simulink model "gm_rgb_gauss_sobel_64bit_full"  (R2022a)
settings: Solver=VariableStepAuto  StartTime=0.0  StopTime=10.0  RelTol=1e-3
undefined symbols (not defined in the file or in its folder): blueMax, blueMin, gray, greenMax, greenMin, redMax, redMin
libraries: hdlsllib x62, visionhdlio x6, visionsources x2
(part 1 of 3)
settings Model: PacingRate=1000  Creator=cxc1831  LastModifiedBy=calvi
settings OptimizationCC: BlockReduction=off  ConditionallyExecuteInputs=off
settings DebuggingCC: ArtificialAlgebraicLoopMsg=none  InheritedTsInSrcMsg=none

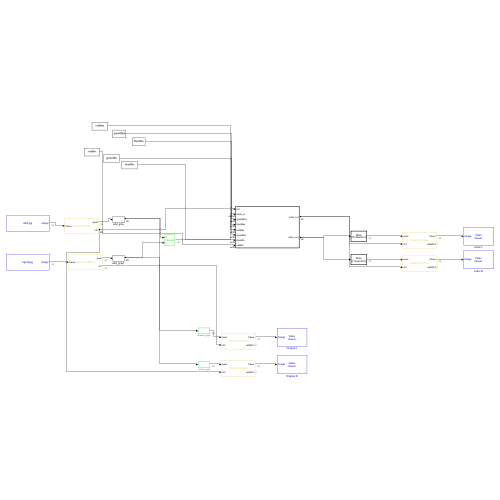
[thumbnail: Simulink's stored preview of the top-level diagram]
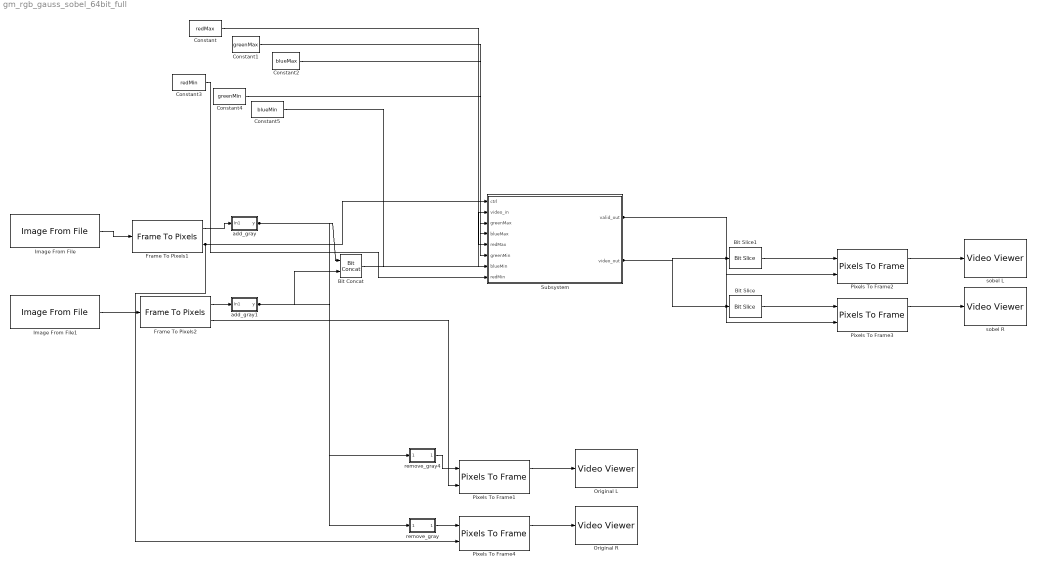
== system gm_rgb_gauss_sobel_64bit_full ==
  Bit Concat : hdlsllib/Logic and Bit Operations/Bit Concat  numInputs=2
  Bit Slice : hdlsllib/Logic and Bit Operations/Bit Slice  lidx=7  ridx=0
      settings: SourceProductBaseCode=SL
  Bit Slice1 : hdlsllib/Logic and Bit Operations/Bit Slice  lidx=15  ridx=8
      settings: SourceProductBaseCode=SL
  Constant : Constant  Value=redMax  OutDataTypeStr=uint8  SampleTime=-1
  Constant1 : Constant  Value=greenMax  OutDataTypeStr=uint8  SampleTime=-1
  Constant2 : Constant  Value=blueMax  OutDataTypeStr=uint8  SampleTime=-1
  Constant3 : Constant  Value=redMin  OutDataTypeStr=uint8  SampleTime=-1  LockScale=on
  Constant4 : Constant  Value=greenMin  OutDataTypeStr=uint8  SampleTime=-1  LockScale=on
  Constant5 : Constant  Value=blueMin  OutDataTypeStr=uint8  SampleTime=-1  LockScale=on
  Frame To Pixels1 : visionhdlio/Frame To Pixels  NumComponents=3  NumPixels=1  VideoFormat=Custom  ActivePixelsPerLine=R  ActiveVideoLines=C  TotalPixelsPerLine=R  TotalVideoLines=C  StartingActiveLine=1  FrontPorch=0  SampleTime=0  VideoFormatCache=Custom  ActivePixelsPerLineCache=R  ActiveVideoLinesCache=C  TotalPixelsPerLineCache=R  TotalVideoLinesCache=C  StartingActiveLineCache=1  FrontPorchCache=0
      settings: SourceProductBaseCode=VT
  Frame To Pixels2 : visionhdlio/Frame To Pixels  NumComponents=3  NumPixels=1  VideoFormat=Custom  ActivePixelsPerLine=R  ActiveVideoLines=C  TotalPixelsPerLine=R  TotalVideoLines=C  StartingActiveLine=1  FrontPorch=0  SampleTime=0  VideoFormatCache=Custom  ActivePixelsPerLineCache=R  ActiveVideoLinesCache=C  TotalPixelsPerLineCache=R  TotalVideoLinesCache=C  StartingActiveLineCache=1  FrontPorchCache=0
      settings: SourceProductBaseCode=VT
  Image From File : visionsources/Image From File  Tag=vipblks_nd  FileName=C:\Projects\ipcore_integration\left3.jpg  Ts=1  imagePorts=One multidimensional signal  OutPortLabels=R|G|B  ImageDataType=Inherit from input image  sdImageDataType=uint(8)  Signed=on  WordLength=16  FractionLengthMode=User-defined  FractionLength=15
  Image From File1 : visionsources/Image From File  Tag=vipblks_nd  FileName=C:\Projects\ipcore_integration\right3.jpg  Ts=1  imagePorts=One multidimensional signal  OutPortLabels=R|G|B  ImageDataType=Inherit from input image  sdImageDataType=uint(8)  Signed=on  WordLength=16  FractionLengthMode=User-defined  FractionLength=15
  Original L : VideoViewer  colormapValue=gray(256)  FigPos=[661 769 562 322]
  Original R : VideoViewer  colormapValue=gray(256)  FigPos=[692 754 485 298]
  Pixels To Frame1 : visionhdlio/Pixels To Frame  NumComponents=3  NumPixels=1  VideoFormat=Custom  ActivePixelsPerLine=R  ActiveVideoLines=C  TotalPixelsPerLine=R  TotalVideoLines=C  VideoFormatCache=Custom  ActivePixelsPerLineCache=R  ActiveVideoLinesCache=C  TotalPixelsPerLineCache=R  TotalVideoLinesCache=C
      settings: SourceProductBaseCode=VT
  Pixels To Frame2 : visionhdlio/Pixels To Frame  NumComponents=1  NumPixels=1  VideoFormat=Custom  ActivePixelsPerLine=R  ActiveVideoLines=C  TotalPixelsPerLine=R  TotalVideoLines=C  VideoFormatCache=Custom  ActivePixelsPerLineCache=R  ActiveVideoLinesCache=C  TotalPixelsPerLineCache=R  TotalVideoLinesCache=C
      settings: SourceProductBaseCode=VT
  Pixels To Frame3 : visionhdlio/Pixels To Frame  NumComponents=1  NumPixels=1  VideoFormat=Custom  ActivePixelsPerLine=R  ActiveVideoLines=C  TotalPixelsPerLine=R  TotalVideoLines=C  VideoFormatCache=Custom  ActivePixelsPerLineCache=R  ActiveVideoLinesCache=C  TotalPixelsPerLineCache=R  TotalVideoLinesCache=C
      settings: SourceProductBaseCode=VT
  Pixels To Frame4 : visionhdlio/Pixels To Frame  NumComponents=3  NumPixels=1  VideoFormat=Custom  ActivePixelsPerLine=R  ActiveVideoLines=C  TotalPixelsPerLine=R  TotalVideoLines=C  VideoFormatCache=Custom  ActivePixelsPerLineCache=R  ActiveVideoLinesCache=C  TotalPixelsPerLineCache=R  TotalVideoLinesCache=C
      settings: SourceProductBaseCode=VT
  Subsystem : Subsystem  TreatAsAtomicUnit=on
  add_gray : Subsystem
  add_gray1 : Subsystem
  remove_gray : Subsystem
  remove_gray4 : Subsystem
  sobel L : VideoViewer  colormapValue=gray(256)  FigPos=[1 1398 2560 1298]
  sobel R : VideoViewer  colormapValue=gray(256)  FigPos=[1 1398 2560 1298]
  wires:
  Constant5/1 -> Subsystem/7(blueMin)
  Constant4/1 -> Subsystem/6(greenMin)
  Constant3/1 -> Subsystem/8(redMin)
  Constant2/1 -> Subsystem/4(blueMax)
  Constant/1 -> Subsystem/5(redMax)
  Constant1/1 -> Subsystem/3(greenMax)
  Subsystem/1(valid_out) -> Pixels To Frame2/2, Pixels To Frame3/2
  Subsystem/2(video_out) -> Bit Slice/1, Bit Slice1/1
  Bit Concat/1 -> Subsystem/2(video_in)
  Bit Slice1/1 -> Pixels To Frame2/1
  Bit Slice/1 -> Pixels To Frame3/1
  Pixels To Frame3/1 -> sobel R/1
  Pixels To Frame2/1 -> sobel L/1
  Pixels To Frame4/1 -> Original R/1
  Pixels To Frame1/1 -> Original L/1
  Frame To Pixels2/1 -> add_gray1/1(In1)
  Frame To Pixels1/1 -> add_gray/1(In1)
  Image From File/1 -> Frame To Pixels1/1
  add_gray1/1(y) -> Bit Concat/2, remove_gray/1(RGB)
  Frame To Pixels1/2 -> Pixels To Frame4/2, Subsystem/1(ctrl)
  remove_gray/1(RGBVector) -> Pixels To Frame4/1
  Image From File1/1 -> Frame To Pixels2/1
  add_gray/1(y) -> Bit Concat/1, remove_gray4/1(RGB)
  remove_gray4/1(RGBVector) -> Pixels To Frame1/1
  Frame To Pixels2/2 -> Pixels To Frame1/2

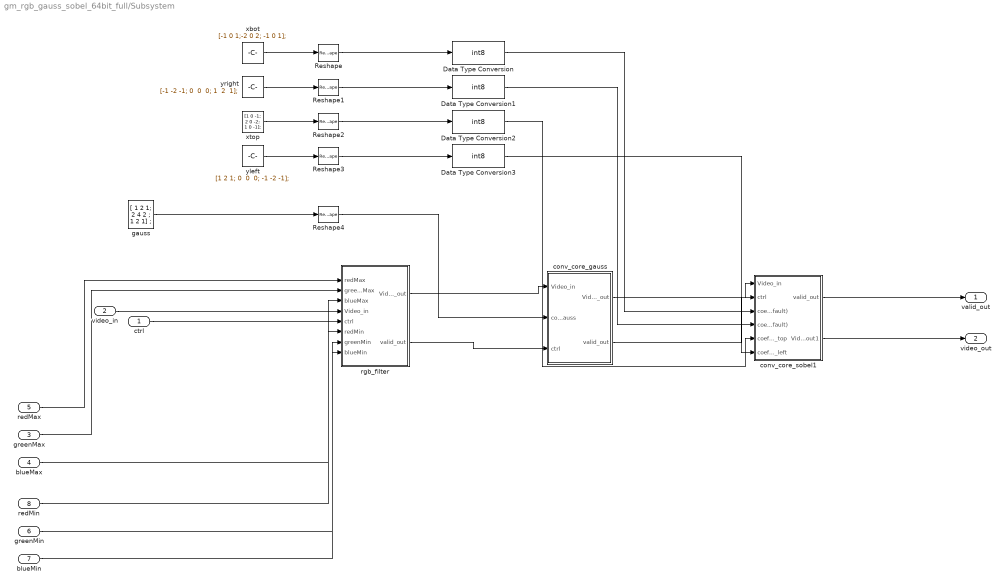
== system gm_rgb_gauss_sobel_64bit_full/Subsystem ==
  ctrl : Inport  SampleTime=2.77039007092199e-06
  video_in : Inport  Port=2  OutDataTypeStr=fixdt(0, 64, 0)  PortDimensions=1  SampleTime=2.77039007092199e-06
  greenMax : Inport  Port=3  OutDataTypeStr=uint8  PortDimensions=1  SampleTime=2.77039007092199e-06
  blueMax : Inport  Port=4  OutDataTypeStr=uint8  PortDimensions=1  SampleTime=2.77039007092199e-06
  redMax : Inport  Port=5  OutDataTypeStr=uint8  PortDimensions=1  SampleTime=2.77039007092199e-06
  greenMin : Inport  Port=6  OutDataTypeStr=uint8  PortDimensions=1  SampleTime=2.77039007092199e-06
  blueMin : Inport  Port=7  OutDataTypeStr=uint8  PortDimensions=1  SampleTime=2.77039007092199e-06
  redMin : Inport  Port=8  OutDataTypeStr=uint8  PortDimensions=1  SampleTime=2.77039007092199e-06
  Data Type Conversion{,1..3} (4 alike) : DataTypeConversion  OutDataTypeStr=int8  SaturateOnIntegerOverflow=off  RndMeth=Floor
  Reshape{,1..4} (5 alike) : Reshape
  conv_core_gauss : Subsystem
  conv_core_sobel1 : Subsystem
  gauss : Constant  Value=|  VectorParams1D=off  OutDataTypeStr=uint8  SampleTime=-1  LockScale=on
      | [ 1  2  1;  2   4   2 ;  1  2  1]
      | ;
  rgb_filter : Subsystem
  xbot : Constant  Value=|  VectorParams1D=off  OutDataTypeStr=int8  SampleTime=-1
      | [-1 0 1;-2 0 2;
      | -1 0 1];
  xtop : Constant  Value=|  VectorParams1D=off  OutDataTypeStr=int8  SampleTime=-1
      | [1 0 -1; 2 0 -2;
      | 1 0 -1];
  yleft : Constant  Value="[1 2 1; 0  0  0; -1 -2 -1];"  VectorParams1D=off  OutDataTypeStr=int8  SampleTime=-1
  yright : Constant  Value=|  VectorParams1D=off  OutDataTypeStr=int8  SampleTime=-1
      | [-1 -2 -1;
      | 0  0  0; 1  2  1];
  valid_out : Outport  SampleTime=2.77039007092199e-06
  video_out : Outport  Port=2  SampleTime=2.77039007092199e-06
  wires:
  ctrl/1 -> rgb_filter/5(ctrl)
  video_in/1 -> rgb_filter/4(Video_in)
  greenMax/1 -> rgb_filter/2(greenMax)
  blueMax/1 -> rgb_filter/3(blueMax)
  redMax/1 -> rgb_filter/1(redMax)
  greenMin/1 -> rgb_filter/7(greenMin)
  blueMin/1 -> rgb_filter/8(blueMin)
  redMin/1 -> rgb_filter/6(redMin)
  Data Type Conversion/1 -> conv_core_sobel1/3(coeffsX_bot(default))
  Data Type Conversion1/1 -> conv_core_sobel1/4(coeffsY_right(default))
  Data Type Conversion2/1 -> conv_core_sobel1/5(coeffsX_top)
  Data Type Conversion3/1 -> conv_core_sobel1/6(coeffsY_left)
  Reshape/1 -> Data Type Conversion/1
  Reshape1/1 -> Data Type Conversion1/1
  Reshape2/1 -> Data Type Conversion2/1
  Reshape3/1 -> Data Type Conversion3/1
  Reshape4/1 -> conv_core_gauss/2(coeffsGauss)
  conv_core_gauss/1(Video_out) -> conv_core_sobel1/1(Video_in)
  conv_core_gauss/2(valid_out) -> conv_core_sobel1/2(ctrl)
  conv_core_sobel1/1(valid_out) -> valid_out/1
  conv_core_sobel1/2(Video_out1) -> video_out/1
  gauss/1 -> Reshape4/1
  rgb_filter/1(Video_out) -> conv_core_gauss/1(Video_in)
  rgb_filter/2(valid_out) -> conv_core_gauss/3(ctrl)
  xbot/1 -> Reshape/1
  xtop/1 -> Reshape2/1
  yleft/1 -> Reshape3/1
  yright/1 -> Reshape1/1

== system gm_rgb_gauss_sobel_64bit_full/add_gray ==
  note: Grayscale = (R * 0.25) + (G * 0.5) + (B * 0.125)
  In1 : Inport
  Bit Concat : hdlsllib/Logic and Bit Operations/Bit Concat  numInputs=4
  Demux : Demux  Outputs=3
  Shift Arithmetic3 : ArithShift  BitShiftNumber=1  BitShiftDirection=Right
  Shift Arithmetic4 : ArithShift  BitShiftNumber=2  BitShiftDirection=Right
  Shift Arithmetic5 : ArithShift  BitShiftNumber=3  BitShiftDirection=Right
  Sum : Sum  Inputs=+++  OutDataTypeStr=uint8
  y : Outport
  wires:
  Shift Arithmetic5/1 -> Sum/3
  Shift Arithmetic3/1 -> Sum/2
  Shift Arithmetic4/1 -> Sum/1
  Sum/1 -> Bit Concat/1
  Demux/3 -> Bit Concat/4, Shift Arithmetic5/1
  Demux/1 -> Bit Concat/2, Shift Arithmetic4/1
  Demux/2 -> Bit Concat/3, Shift Arithmetic3/1
  In1/1 -> Demux/1
  Bit Concat/1 -> y/1

== system gm_rgb_gauss_sobel_64bit_full/add_gray1 ==
  note: Grayscale = (R * 0.25) + (G * 0.5) + (B * 0.125)
  In1 : Inport
  Bit Concat : hdlsllib/Logic and Bit Operations/Bit Concat  numInputs=4
  Demux : Demux  Outputs=3
  Shift Arithmetic3 : ArithShift  BitShiftNumber=1  BitShiftDirection=Right
  Shift Arithmetic4 : ArithShift  BitShiftNumber=2  BitShiftDirection=Right
  Shift Arithmetic5 : ArithShift  BitShiftNumber=3  BitShiftDirection=Right
  Sum : Sum  Inputs=+++  OutDataTypeStr=uint8
  y : Outport
  wires:
  Shift Arithmetic5/1 -> Sum/3
  Shift Arithmetic3/1 -> Sum/2
  Shift Arithmetic4/1 -> Sum/1
  Sum/1 -> Bit Concat/1
  Demux/3 -> Bit Concat/4, Shift Arithmetic5/1
  Demux/1 -> Bit Concat/2, Shift Arithmetic4/1
  Demux/2 -> Bit Concat/3, Shift Arithmetic3/1
  In1/1 -> Demux/1
  Bit Concat/1 -> y/1

== system gm_rgb_gauss_sobel_64bit_full/remove_gray ==
  note: RGB represented in
      | 32'hFFRRGGBB
  RGB : Inport
  Bit Slice : hdlsllib/Logic and Bit Operations/Bit Slice  lidx=23  ridx=16
      settings: SourceProductBaseCode=SL
  Bit Slice1 : hdlsllib/Logic and Bit Operations/Bit Slice  lidx=15  ridx=8
      settings: SourceProductBaseCode=SL
  Bit Slice2 : hdlsllib/Logic and Bit Operations/Bit Slice  lidx=7  ridx=0
      settings: SourceProductBaseCode=SL
  Mux : Mux  Inputs=3
  Signal Specification : SignalSpecification
  Transpose : Math  Operator=transpose  SignedPower=on
  RGBVector : Outport  VectorParamsAs1DForOutWhenUnconnected=off
  wires:
  Mux/1 -> Transpose/1
  Bit Slice/1 -> Mux/1
  Bit Slice2/1 -> Mux/3
  Bit Slice1/1 -> Mux/2
  RGB/1 -> Bit Slice2/1, Bit Slice1/1, Bit Slice/1
  Transpose/1 -> Signal Specification/1
  Signal Specification/1 -> RGBVector/1

== system gm_rgb_gauss_sobel_64bit_full/remove_gray4 ==
  note: RGB represented in
      | 32'hFFRRGGBB
  RGB : Inport
  Bit Slice : hdlsllib/Logic and Bit Operations/Bit Slice  lidx=23  ridx=16
      settings: SourceProductBaseCode=SL
  Bit Slice1 : hdlsllib/Logic and Bit Operations/Bit Slice  lidx=15  ridx=8
      settings: SourceProductBaseCode=SL
  Bit Slice2 : hdlsllib/Logic and Bit Operations/Bit Slice  lidx=7  ridx=0
      settings: SourceProductBaseCode=SL
  Mux : Mux  Inputs=3
  Signal Specification : SignalSpecification
  Transpose : Math  Operator=transpose  SignedPower=on
  RGBVector : Outport  VectorParamsAs1DForOutWhenUnconnected=off
  wires:
  Mux/1 -> Transpose/1
  Bit Slice/1 -> Mux/1
  Bit Slice2/1 -> Mux/3
  Bit Slice1/1 -> Mux/2
  RGB/1 -> Bit Slice2/1, Bit Slice1/1, Bit Slice/1
  Transpose/1 -> Signal Specification/1
  Signal Specification/1 -> RGBVector/1

== system gm_rgb_gauss_sobel_64bit_full/Subsystem/conv_core_gauss ==
  Video_in : Inport  OutDataTypeStr=fixdt(0, 64, 0)  PortDimensions=1  SampleTime=2.77039007092199e-06
  coeffsGauss : Inport  Port=2  OutDataTypeStr=uint8  PortDimensions=[9]  SampleTime=2.77039007092199e-06
  ctrl : Inport  Port=3  SampleTime=2.77039007092199e-06
  Bus Selector : BusSelector  OutputSignals=valid
  Delay1 : Delay  InitialCondition=0
  Subsystem1 : Subsystem
  Video_out : Outport  SampleTime=2.77039007092199e-06  VectorParamsAs1DForOutWhenUnconnected=off
  valid_out : Outport  Port=2  SampleTime=2.77039007092199e-06  VectorParamsAs1DForOutWhenUnconnected=off
  wires:
  Video_in/1 -> Subsystem1/1(VideoIn)
  coeffsGauss/1 -> Subsystem1/2(coeffsGauss)
  ctrl/1 -> Bus Selector/1, Delay1/1
  Bus Selector/1 -> Subsystem1/3(Enable)
  Delay1/1 -> valid_out/1
  Subsystem1/1(Video_out) -> Video_out/1

== system gm_rgb_gauss_sobel_64bit_full/Subsystem/conv_core_sobel1 ==
  Video_in : Inport  OutDataTypeStr=fixdt(0, 64, 0)  PortDimensions=1  SampleTime=2.77039007092199e-06
  ctrl : Inport  Port=2  SampleTime=2.77039007092199e-06
  coeffsX_bot(default) : Inport  Port=3  OutDataTypeStr=int8  PortDimensions=[9]  SampleTime=2.77039007092199e-06
  coeffsY_right(default) : Inport  Port=4  OutDataTypeStr=int8  PortDimensions=[9]  SampleTime=2.77039007092199e-06
  coeffsX_top : Inport  Port=5  OutDataTypeStr=int8  PortDimensions=[9]  SampleTime=2.77039007092199e-06
  coeffsY_left : Inport  Port=6  OutDataTypeStr=int8  PortDimensions=[9]  SampleTime=2.77039007092199e-06
  Bit Concat1 : hdlsllib/Logic and Bit Operations/Bit Concat  numInputs=2
  Bus Selector : BusSelector  OutputSignals=valid
  Delay1 : Delay  InitialCondition=0
  Subsystem1 : Subsystem
  valid_out : Outport  SampleTime=2.77039007092199e-06  VectorParamsAs1DForOutWhenUnconnected=off
  Video_out1 : Outport  Port=2  SampleTime=2.77039007092199e-06  VectorParamsAs1DForOutWhenUnconnected=off
  wires:
  Video_in/1 -> Subsystem1/1(vidIn)
  ctrl/1 -> Bus Selector/1, Delay1/1
  coeffsX_bot(default)/1 -> Subsystem1/2(coeffsX_bot(default))
  coeffsY_right(default)/1 -> Subsystem1/3(coeffsY_bot(default))
  coeffsX_top/1 -> Subsystem1/4(coeffsX_Top)
  coeffsY_left/1 -> Subsystem1/5(coeffsY_Left)
  Bit Concat1/1 -> Video_out1/1
  Bus Selector/1 -> Subsystem1/6(Enable)
  Delay1/1 -> valid_out/1
  Subsystem1/1(sobel R) -> Bit Concat1/2
  Subsystem1/2(sobel L) -> Bit Concat1/1

== system gm_rgb_gauss_sobel_64bit_full/Subsystem/rgb_filter ==
  redMax : Inport  OutDataTypeStr=uint8  PortDimensions=1  SampleTime=2.77039007092199e-06
  greenMax : Inport  Port=2  OutDataTypeStr=uint8  PortDimensions=1  SampleTime=2.77039007092199e-06
  blueMax : Inport  Port=3  OutDataTypeStr=uint8  PortDimensions=1  SampleTime=2.77039007092199e-06
  Video_in : Inport  Port=4  OutDataTypeStr=fixdt(0, 64, 0)  PortDimensions=1  SampleTime=2.77039007092199e-06
  ctrl : Inport  Port=5  SampleTime=2.77039007092199e-06
  redMin : Inport  Port=6  OutDataTypeStr=uint8  PortDimensions=1  SampleTime=2.77039007092199e-06
  greenMin : Inport  Port=7  OutDataTypeStr=uint8  PortDimensions=1  SampleTime=2.77039007092199e-06
  blueMin : Inport  Port=8  OutDataTypeStr=uint8  PortDimensions=1  SampleTime=2.77039007092199e-06
  Bit Concat1 : hdlsllib/Logic and Bit Operations/Bit Concat  numInputs=2
  Bus Selector : BusSelector  OutputSignals=valid
  Delay1 : Delay  DelayLength=1  InitialCondition=0
  Subsystem1 : Subsystem
  Video_out : Outport  SampleTime=2.77039007092199e-06  VectorParamsAs1DForOutWhenUnconnected=off
  valid_out : Outport  Port=2  SampleTime=2.77039007092199e-06  VectorParamsAs1DForOutWhenUnconnected=off
  wires:
  redMax/1 -> Subsystem1/2(redmax)
  greenMax/1 -> Subsystem1/3(greenmax)
  blueMax/1 -> Subsystem1/4(bluemax)
  Video_in/1 -> Subsystem1/1(In2)
  ctrl/1 -> Bus Selector/1, Delay1/1
  redMin/1 -> Subsystem1/5(redMin)
  greenMin/1 -> Subsystem1/6(greenMin)
  blueMin/1 -> Subsystem1/7(blueMin)
  Bit Concat1/1 -> Video_out/1
  Bus Selector/1 -> Subsystem1/8(Enable)
  Delay1/1 -> valid_out/1
  Subsystem1/1(Video_outLeft) -> Bit Concat1/1
  Subsystem1/2(Video_outRight) -> Bit Concat1/2

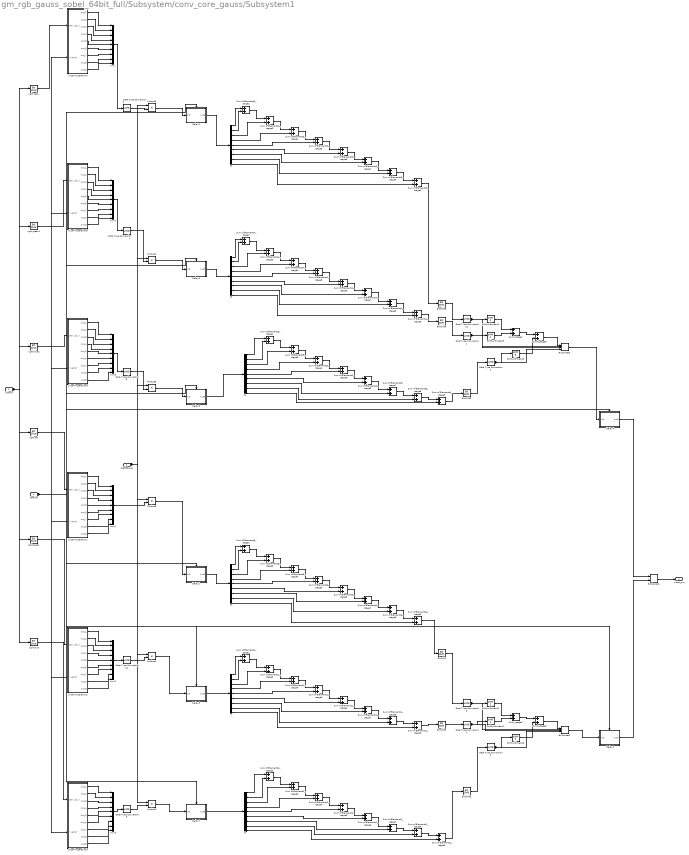
== system gm_rgb_gauss_sobel_64bit_full/Subsystem/conv_core_gauss/Subsystem1 ==
  VideoIn : Inport  OutDataTypeStr=fixdt(0, 64, 0)  PortDimensions=1  SampleTime=2.77039007092199e-06
  coeffsGauss : Inport  Port=2  OutDataTypeStr=uint8  PortDimensions=[9]  SampleTime=2.77039007092199e-06
  Enable : Inport  Port=3  OutDataTypeStr=boolean  SampleTime=2.77039007092199e-06
  Bit Concat1 : hdlsllib/Logic and Bit Operations/Bit Concat  numInputs=2
  Bit Concat2 : hdlsllib/Logic and Bit Operations/Bit Concat  numInputs=4
  Bit Concat3 : hdlsllib/Logic and Bit Operations/Bit Concat  numInputs=4
  Bit Shift{,1..5} (6 alike) : hdlsllib/Logic and Bit Operations/Bit Shift  mode=Shift Right Arithmetic  N=double(4)
  Data Type Conversion{1..10,12} (11 alike) : DataTypeConversion  OutDataTypeStr=uint8  SampleTime=2.77039007092199e-06  SaturateOnIntegerOverflow=off  RndMeth=Floor
  Delay1 : Subsystem
      settings: MinAlgLoopOccurrences=on
  Delay2 : Subsystem
      settings: MinAlgLoopOccurrences=on
  Delay3 : Subsystem
      settings: MinAlgLoopOccurrences=on
  Delay4 : Subsystem
      settings: MinAlgLoopOccurrences=on
  Delay5 : Subsystem
      settings: MinAlgLoopOccurrences=on
  Delay6 : Subsystem
      settings: MinAlgLoopOccurrences=on
  Delay7 : Subsystem
      settings: MinAlgLoopOccurrences=on
  Delay8 : Subsystem
      settings: MinAlgLoopOccurrences=on
  Product{1..6} (6 alike) : Product  Inputs=**  OutDataTypeStr=uint16  SaturateOnIntegerOverflow=on  SampleTime=2.77039007092199e-06
  Shift Arithmetic1 : ArithShift  BitShiftNumber=1  BinPtShiftNumber=double(0)
  Shift Arithmetic2 : ArithShift  BitShiftNumber=2  BinPtShiftNumber=double(0)
  Shift Arithmetic3 : ArithShift  BitShiftNumber=1  BinPtShiftNumber=double(0)
  Shift Arithmetic4 : ArithShift  BitShiftNumber=2  BinPtShiftNumber=double(0)
  Shift Arithmetic5 : ArithShift  BitShiftNumber=3  BinPtShiftNumber=double(0)
  Shift Arithmetic6 : ArithShift  BitShiftNumber=3  BinPtShiftNumber=double(0)
  Sum of Elements1_stage{2..9} (8 alike) : Sum  AccumDataTypeStr=uint32  OutDataTypeStr=uint32  SaturateOnIntegerOverflow=on  SampleTime=2.77039007092199e-06
  Sum of Elements2_stage{2..9} (8 alike) : Sum  AccumDataTypeStr=uint32  OutDataTypeStr=uint32  SaturateOnIntegerOverflow=on  SampleTime=2.77039007092199e-06
  Sum of Elements3_stage{2..9} (8 alike) : Sum  AccumDataTypeStr=uint32  OutDataTypeStr=uint32  SaturateOnIntegerOverflow=on  SampleTime=2.77039007092199e-06
  Sum of Elements4_stage{2..9} (8 alike) : Sum  AccumDataTypeStr=uint32  OutDataTypeStr=uint32  SaturateOnIntegerOverflow=on  SampleTime=2.77039007092199e-06
  Sum of Elements5_stage{2..9} (8 alike) : Sum  AccumDataTypeStr=uint32  OutDataTypeStr=uint32  SaturateOnIntegerOverflow=on  SampleTime=2.77039007092199e-06
  Sum of Elements6_stage{2..9} (8 alike) : Sum  AccumDataTypeStr=uint32  OutDataTypeStr=uint32  SaturateOnIntegerOverflow=on  SampleTime=2.77039007092199e-06
  Sum1_stage2 : Sum  AccumDataTypeStr=uint8  OutDataTypeStr=uint8  SampleTime=2.77039007092199e-06
  Sum1_stage3 : Sum  AccumDataTypeStr=uint8  OutDataTypeStr=uint8  SampleTime=2.77039007092199e-06
  Sum2_stage2 : Sum  AccumDataTypeStr=uint8  OutDataTypeStr=uint8  SampleTime=2.77039007092199e-06
  Sum2_stage3 : Sum  AccumDataTypeStr=uint8  OutDataTypeStr=uint8  SampleTime=2.77039007092199e-06
  mux{,1..5} (6 alike) : Mux  Inputs=9
  right blue : hdlsllib/Logic and Bit Operations/Bit Slice  lidx=double(7)  ridx=double(0)
      settings: SourceProductBaseCode=SL
  right blue1 : hdlsllib/Logic and Bit Operations/Bit Slice  lidx=double(39)  ridx=double(32)
      settings: SourceProductBaseCode=SL
  right green : hdlsllib/Logic and Bit Operations/Bit Slice  lidx=double(15)  ridx=double(8)
      settings: SourceProductBaseCode=SL
  right green1 : hdlsllib/Logic and Bit Operations/Bit Slice  lidx=double(47)  ridx=double(40)
      settings: SourceProductBaseCode=SL
  right red : hdlsllib/Logic and Bit Operations/Bit Slice  lidx=double(23)  ridx=double(16)
      settings: SourceProductBaseCode=SL
  right red1 : hdlsllib/Logic and Bit Operations/Bit Slice  lidx=double(55)  ridx=double(48)
      settings: SourceProductBaseCode=SL
  slicer R operation1 : Subsystem
  slicer R operation2 : Subsystem
  slicer R operation3 : Subsystem
  slicer R operation4 : Subsystem
  slicer R operation5 : Subsystem
  slicer R operation6 : Subsystem
  t{,1..5} (6 alike) : Demux  Outputs=9
  Video_out : Outport  SampleTime=2.77039007092199e-06  InitialOutput=0  VectorParamsAs1DForOutWhenUnconnected=off
  wires:
  Enable/1 -> Delay8/Enable, Delay7/Enable, Delay6/Enable, Delay5/Enable, Delay4/Enable, Delay3/Enable, Delay2/Enable, Delay1/Enable, slicer R operation6/2(<valid>), slicer R operation5/2(<valid>), slicer R operation4/2(<valid>), slicer R operation3/2(<valid>), slicer R operation2/2(<valid>), slicer R operation1/2(<valid>)
  VideoIn/1 -> right red1/1, right red/1, right green1/1, right green/1, right blue1/1, right blue/1
  coeffsGauss/1 -> Product6/1, Product5/1, Product4/1, Product3/1, Product2/1, Product1/1
  Bit Concat1/1 -> Video_out/1
  Bit Concat2/1 -> Delay3/1(in0)
  Bit Concat3/1 -> Delay4/1(in0)
  Bit Shift/1 -> Data Type Conversion5/1
  Bit Shift1/1 -> Data Type Conversion4/1
  Bit Shift2/1 -> Data Type Conversion3/1
  Bit Shift3/1 -> Data Type Conversion12/1
  Bit Shift4/1 -> Data Type Conversion1/1
  Bit Shift5/1 -> Data Type Conversion2/1
  Data Type Conversion1/1 -> Shift Arithmetic3/1, Bit Concat3/3
  Data Type Conversion10/1 -> Product1/2
  Data Type Conversion12/1 -> Shift Arithmetic4/1, Bit Concat3/2
  Data Type Conversion2/1 -> Shift Arithmetic5/1, Bit Concat3/4
  Data Type Conversion3/1 -> Shift Arithmetic6/1, Bit Concat2/4
  Data Type Conversion4/1 -> Shift Arithmetic1/1, Bit Concat2/3
  Data Type Conversion5/1 -> Shift Arithmetic2/1, Bit Concat2/2
  Data Type Conversion6/1 -> Product3/2
  Data Type Conversion7/1 -> Product4/2
  Data Type Conversion8/1 -> Product5/2
  Data Type Conversion9/1 -> Product2/2
  Delay1/1(out0) -> t5/1
  Delay2/1(out0) -> t2/1
  Delay3/1(out0) -> Bit Concat1/2
  Delay4/1(out0) -> Bit Concat1/1
  Delay5/1(out0) -> t/1
  Delay6/1(out0) -> t3/1
  Delay7/1(out0) -> t1/1
  Delay8/1(out0) -> t4/1
  mux/1 -> Data Type Conversion6/1
  mux1/1 -> Product6/2
  mux2/1 -> Data Type Conversion10/1
  mux3/1 -> Data Type Conversion9/1
  mux4/1 -> Data Type Conversion7/1
  mux5/1 -> Data Type Conversion8/1
  Product1/1 -> Delay5/1(in0)
  Product2/1 -> Delay7/1(in0)
  Product3/1 -> Delay2/1(in0)
  Product4/1 -> Delay6/1(in0)
  Product5/1 -> Delay8/1(in0)
  Product6/1 -> Delay1/1(in0)
  Shift Arithmetic1/1 -> Sum1_stage2/2
  Shift Arithmetic2/1 -> Sum1_stage2/1
  Shift Arithmetic3/1 -> Sum2_stage2/2
  Shift Arithmetic4/1 -> Sum2_stage2/1
  Shift Arithmetic5/1 -> Sum2_stage3/2
  Shift Arithmetic6/1 -> Sum1_stage3/2
  Sum1_stage3/1 -> Bit Concat2/1
  Sum2_stage3/1 -> Bit Concat3/1
  right blue/1 -> slicer R operation3/1(channel_in)
  right blue1/1 -> slicer R operation6/1(channel_in)
  right green/1 -> slicer R operation2/1(channel_in)
  right green1/1 -> slicer R operation5/1(channel_in)
  right red/1 -> slicer R operation1/1(channel_in)
  right red1/1 -> slicer R operation4/1(channel_in)
  slicer R operation1/1(out_1) -> mux1/1
  slicer R operation1/2(out_2) -> mux1/2
  slicer R operation1/3(out_3) -> mux1/3
  slicer R operation1/4(out_4) -> mux1/4
  slicer R operation1/5(out_5) -> mux1/5
  slicer R operation1/6(out_6) -> mux1/6
  slicer R operation1/7(out_7) -> mux1/7
  slicer R operation1/8(out_8) -> mux1/8
  slicer R operation1/9(out_9) -> mux1/9
  slicer R operation2/1(out_1) -> mux2/1
  slicer R operation2/2(out_2) -> mux2/2
  slicer R operation2/3(out_3) -> mux2/3
  slicer R operation2/4(out_4) -> mux2/4
  slicer R operation2/5(out_5) -> mux2/5
  slicer R operation2/6(out_6) -> mux2/6
  slicer R operation2/7(out_7) -> mux2/7
  slicer R operation2/8(out_8) -> mux2/8
  slicer R operation2/9(out_9) -> mux2/9
  slicer R operation3/1(out_1) -> mux3/1
  slicer R operation3/2(out_2) -> mux3/2
  slicer R operation3/3(out_3) -> mux3/3
  slicer R operation3/4(out_4) -> mux3/4
  slicer R operation3/5(out_5) -> mux3/5
  slicer R operation3/6(out_6) -> mux3/6
  slicer R operation3/7(out_7) -> mux3/7
  slicer R operation3/8(out_8) -> mux3/8
  slicer R operation3/9(out_9) -> mux3/9
  slicer R operation4/1(out_1) -> mux/1
  slicer R operation4/2(out_2) -> mux/2
  slicer R operation4/3(out_3) -> mux/3
  slicer R operation4/4(out_4) -> mux/4
  slicer R operation4/5(out_5) -> mux/5
  slicer R operation4/6(out_6) -> mux/6
  slicer R operation4/7(out_7) -> mux/7
  slicer R operation4/8(out_8) -> mux/8
  slicer R operation4/9(out_9) -> mux/9
  slicer R operation5/1(out_1) -> mux4/1
  slicer R operation5/2(out_2) -> mux4/2
  slicer R operation5/3(out_3) -> mux4/3
  slicer R operation5/4(out_4) -> mux4/4
  slicer R operation5/5(out_5) -> mux4/5
  slicer R operation5/6(out_6) -> mux4/6
  slicer R operation5/7(out_7) -> mux4/7
  slicer R operation5/8(out_8) -> mux4/8
  slicer R operation5/9(out_9) -> mux4/9
  slicer R operation6/1(out_1) -> mux5/1
  slicer R operation6/2(out_2) -> mux5/2
  slicer R operation6/3(out_3) -> mux5/3
  slicer R operation6/4(out_4) -> mux5/4
  slicer R operation6/5(out_5) -> mux5/5
  slicer R operation6/6(out_6) -> mux5/6
  slicer R operation6/7(out_7) -> mux5/7
  slicer R operation6/8(out_8) -> mux5/8
  slicer R operation6/9(out_9) -> mux5/9
  Sum1_stage2/1 -> Sum1_stage3/1
  Sum2_stage2/1 -> Sum2_stage3/1
  Sum of Elements1_stage9/1 -> Bit Shift1/1
  t/1 -> Sum of Elements1_stage2/1
  t/2 -> Sum of Elements1_stage2/2
  t/3 -> Sum of Elements1_stage3/2
  t/4 -> Sum of Elements1_stage4/2
  t/5 -> Sum of Elements1_stage5/2
  t/6 -> Sum of Elements1_stage6/2
  t/7 -> Sum of Elements1_stage7/2
  t/8 -> Sum of Elements1_stage8/2
  t/9 -> Sum of Elements1_stage9/2
  Sum of Elements1_stage2/1 -> Sum of Elements1_stage3/1
  Sum of Elements1_stage3/1 -> Sum of Elements1_stage4/1
  Sum of Elements1_stage4/1 -> Sum of Elements1_stage5/1
  Sum of Elements1_stage5/1 -> Sum of Elements1_stage6/1
  Sum of Elements1_stage6/1 -> Sum of Elements1_stage7/1
  Sum of Elements1_stage7/1 -> Sum of Elements1_stage8/1
  Sum of Elements1_stage8/1 -> Sum of Elements1_stage9/1
  Sum of Elements2_stage9/1 -> Bit Shift2/1
  t1/1 -> Sum of Elements2_stage2/1
  t1/2 -> Sum of Elements2_stage2/2
  t1/3 -> Sum of Elements2_stage3/2
  t1/4 -> Sum of Elements2_stage4/2
  t1/5 -> Sum of Elements2_stage5/2
  t1/6 -> Sum of Elements2_stage6/2
  t1/7 -> Sum of Elements2_stage7/2
  t1/8 -> Sum of Elements2_stage8/2
  t1/9 -> Sum of Elements2_stage9/2
  Sum of Elements2_stage2/1 -> Sum of Elements2_stage3/1
  Sum of Elements2_stage3/1 -> Sum of Elements2_stage4/1
  Sum of Elements2_stage4/1 -> Sum of Elements2_stage5/1
  Sum of Elements2_stage5/1 -> Sum of Elements2_stage6/1
  Sum of Elements2_stage6/1 -> Sum of Elements2_stage7/1
  Sum of Elements2_stage7/1 -> Sum of Elements2_stage8/1
  Sum of Elements2_stage8/1 -> Sum of Elements2_stage9/1
  Sum of Elements3_stage9/1 -> Bit Shift3/1
  t2/1 -> Sum of Elements3_stage2/1
  t2/2 -> Sum of Elements3_stage2/2
  t2/3 -> Sum of Elements3_stage3/2
  t2/4 -> Sum of Elements3_stage4/2
  t2/5 -> Sum of Elements3_stage5/2
  t2/6 -> Sum of Elements3_stage6/2
  t2/7 -> Sum of Elements3_stage7/2
  t2/8 -> Sum of Elements3_stage8/2
  t2/9 -> Sum of Elements3_stage9/2
  Sum of Elements3_stage2/1 -> Sum of Elements3_stage3/1
  Sum of Elements3_stage3/1 -> Sum of Elements3_stage4/1
  Sum of Elements3_stage4/1 -> Sum of Elements3_stage5/1
  Sum of Elements3_stage5/1 -> Sum of Elements3_stage6/1
  Sum of Elements3_stage6/1 -> Sum of Elements3_stage7/1
  Sum of Elements3_stage7/1 -> Sum of Elements3_stage8/1
  Sum of Elements3_stage8/1 -> Sum of Elements3_stage9/1
  Sum of Elements4_stage9/1 -> Bit Shift4/1
  t3/1 -> Sum of Elements4_stage2/1
  t3/2 -> Sum of Elements4_stage2/2
  t3/3 -> Sum of Elements4_stage3/2
  t3/4 -> Sum of Elements4_stage4/2
  t3/5 -> Sum of Elements4_stage5/2
  t3/6 -> Sum of Elements4_stage6/2
  t3/7 -> Sum of Elements4_stage7/2
  t3/8 -> Sum of Elements4_stage8/2
  t3/9 -> Sum of Elements4_stage9/2
  Sum of Elements4_stage2/1 -> Sum of Elements4_stage3/1
  Sum of Elements4_stage3/1 -> Sum of Elements4_stage4/1
  Sum of Elements4_stage4/1 -> Sum of Elements4_stage5/1
  Sum of Elements4_stage5/1 -> Sum of Elements4_stage6/1
  Sum of Elements4_stage6/1 -> Sum of Elements4_stage7/1
  Sum of Elements4_stage7/1 -> Sum of Elements4_stage8/1
  Sum of Elements4_stage8/1 -> Sum of Elements4_stage9/1
  Sum of Elements5_stage9/1 -> Bit Shift5/1
  t4/1 -> Sum of Elements5_stage2/1
  t4/2 -> Sum of Elements5_stage2/2
  t4/3 -> Sum of Elements5_stage3/2
  t4/4 -> Sum of Elements5_stage4/2
  t4/5 -> Sum of Elements5_stage5/2
  t4/6 -> Sum of Elements5_stage6/2
  t4/7 -> Sum of Elements5_stage7/2
  t4/8 -> Sum of Elements5_stage8/2
  t4/9 -> Sum of Elements5_stage9/2
  Sum of Elements5_stage2/1 -> Sum of Elements5_stage3/1
  Sum of Elements5_stage3/1 -> Sum of Elements5_stage4/1
  Sum of Elements5_stage4/1 -> Sum of Elements5_stage5/1
  Sum of Elements5_stage5/1 -> Sum of Elements5_stage6/1
  Sum of Elements5_stage6/1 -> Sum of Elements5_stage7/1
  Sum of Elements5_stage7/1 -> Sum of Elements5_stage8/1
  Sum of Elements5_stage8/1 -> Sum of Elements5_stage9/1
  Sum of Elements6_stage9/1 -> Bit Shift/1
  t5/1 -> Sum of Elements6_stage2/1
  t5/2 -> Sum of Elements6_stage2/2
  t5/3 -> Sum of Elements6_stage3/2
  t5/4 -> Sum of Elements6_stage4/2
  t5/5 -> Sum of Elements6_stage5/2
  t5/6 -> Sum of Elements6_stage6/2
  t5/7 -> Sum of Elements6_stage7/2
  t5/8 -> Sum of Elements6_stage8/2
  t5/9 -> Sum of Elements6_stage9/2
  Sum of Elements6_stage2/1 -> Sum of Elements6_stage3/1
  Sum of Elements6_stage3/1 -> Sum of Elements6_stage4/1
  Sum of Elements6_stage4/1 -> Sum of Elements6_stage5/1
  Sum of Elements6_stage5/1 -> Sum of Elements6_stage6/1
  Sum of Elements6_stage6/1 -> Sum of Elements6_stage7/1
  Sum of Elements6_stage7/1 -> Sum of Elements6_stage8/1
  Sum of Elements6_stage8/1 -> Sum of Elements6_stage9/1

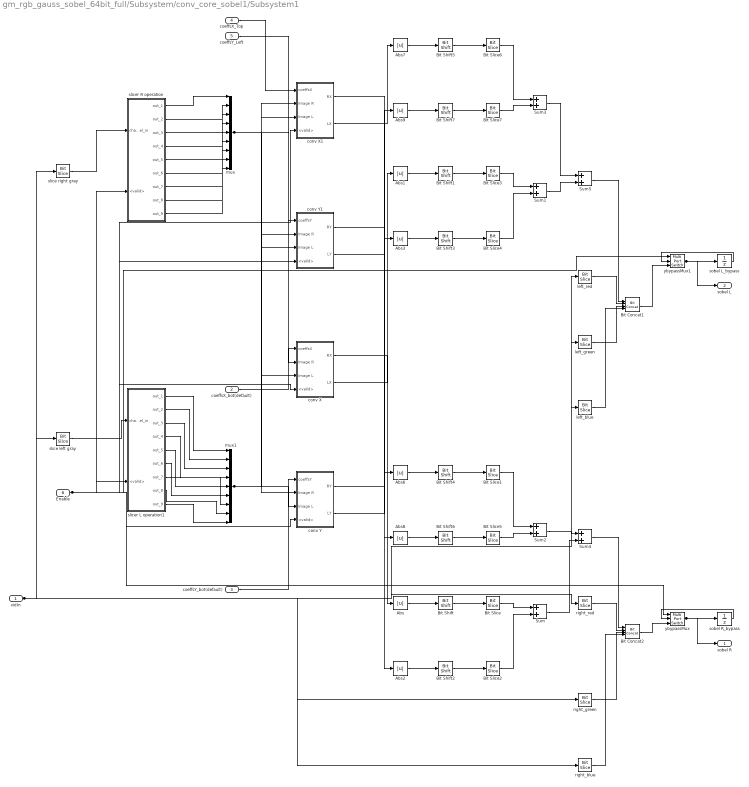
== system gm_rgb_gauss_sobel_64bit_full/Subsystem/conv_core_sobel1/Subsystem1 ==
  vidIn : Inport  OutDataTypeStr=fixdt(0, 64, 0)  PortDimensions=1  SampleTime=2.77039007092199e-06
  coeffsX_bot(default) : Inport  Port=2  OutDataTypeStr=int8  PortDimensions=[9]  SampleTime=2.77039007092199e-06
  coeffsY_bot(default) : Inport  Port=3  OutDataTypeStr=int8  PortDimensions=[9]  SampleTime=2.77039007092199e-06
  coeffsX_Top : Inport  Port=4  OutDataTypeStr=int8  PortDimensions=[9]  SampleTime=2.77039007092199e-06
  coeffsY_Left : Inport  Port=5  OutDataTypeStr=int8  PortDimensions=[9]  SampleTime=2.77039007092199e-06
  Enable : Inport  Port=6  OutDataTypeStr=boolean  SampleTime=2.77039007092199e-06
  Abs{,1..3,6..9} (8 alike) : Abs  SampleTime=2.77039007092199e-06  OutDataTypeStr=uint8  SaturateOnIntegerOverflow=off
  Bit Concat1 : hdlsllib/Logic and Bit Operations/Bit Concat  numInputs=4
  Bit Concat2 : hdlsllib/Logic and Bit Operations/Bit Concat  numInputs=4
  Bit Shift{,1..7} (8 alike) : hdlsllib/Logic and Bit Operations/Bit Shift  mode=Shift Right Logical  N=double(1)
  Bit Slice{,1..7} (8 alike) : hdlsllib/Logic and Bit Operations/Bit Slice  lidx=double(6)  ridx=double(0)
      settings: SourceProductBaseCode=SL
  Sum{,1..3} (4 alike) : Sum  AccumDataTypeStr=uint32  OutDataTypeStr=uint8  SampleTime=2.77039007092199e-06
  Sum4 : Sum  AccumDataTypeStr=uint8  OutDataTypeStr=uint8  SampleTime=2.77039007092199e-06
  Sum5 : Sum  AccumDataTypeStr=uint8  OutDataTypeStr=uint8  SampleTime=2.77039007092199e-06
  conv X : Subsystem
  conv X1 : Subsystem
  conv Y : Subsystem
  conv Y1 : Subsystem
  left_blue : hdlsllib/Logic and Bit Operations/Bit Slice  lidx=double(39)  ridx=double(32)
      settings: SourceProductBaseCode=SL
  left_green : hdlsllib/Logic and Bit Operations/Bit Slice  lidx=double(47)  ridx=double(40)
      settings: SourceProductBaseCode=SL
  left_red : hdlsllib/Logic and Bit Operations/Bit Slice  lidx=double(55)  ridx=double(48)
      settings: SourceProductBaseCode=SL
  mux : Mux  Inputs=9
  mux1 : Mux  Inputs=9
  right_blue : hdlsllib/Logic and Bit Operations/Bit Slice  lidx=double(7)  ridx=double(0)
      settings: SourceProductBaseCode=SL
  right_green : hdlsllib/Logic and Bit Operations/Bit Slice  lidx=double(15)  ridx=double(8)
      settings: SourceProductBaseCode=SL
  right_red : hdlsllib/Logic and Bit Operations/Bit Slice  lidx=double(23)  ridx=double(16)
      settings: SourceProductBaseCode=SL
  slice left gray : hdlsllib/Logic and Bit Operations/Bit Slice  lidx=double(63)  ridx=double(56)
      settings: SourceProductBaseCode=SL
  slice right gray : hdlsllib/Logic and Bit Operations/Bit Slice  lidx=double(31)  ridx=double(24)
      settings: SourceProductBaseCode=SL
  slicer L operation1 : Subsystem
  slicer R operation : Subsystem
  sobel L_bypass : UnitDelay  SampleTime=2.77039007092199e-06
  sobel R_bypass : UnitDelay  SampleTime=2.77039007092199e-06
  ybypassMux : MultiPortSwitch  DataPortOrder=Zero-based contiguous  Inputs=2  zeroidx=on  OutDataTypeStr=uint32  SampleTime=2.77039007092199e-06  SaturateOnIntegerOverflow=off  InputSameDT=off
  ybypassMux1 : MultiPortSwitch  DataPortOrder=Zero-based contiguous  Inputs=2  zeroidx=on  OutDataTypeStr=uint32  SampleTime=2.77039007092199e-06  SaturateOnIntegerOverflow=off  InputSameDT=off
  sobel R : Outport  SampleTime=2.77039007092199e-06  InitialOutput=0
  sobel L : Outport  Port=2  SampleTime=2.77039007092199e-06  InitialOutput=0
  wires:
  Enable/1 -> ybypassMux1/1, ybypassMux/1, slicer R operation/2(<valid>), slicer L operation1/2(<valid>), conv Y1/4(<valid>), conv Y/4(<valid>), conv X1/4(<valid>), conv X/4(<valid>)
  vidIn/1 -> slice right gray/1, slice left gray/1, right_red/1, right_green/1, right_blue/1, left_red/1, left_green/1, left_blue/1
  coeffsX_bot(default)/1 -> conv X/1(coeffsX)
  coeffsY_bot(default)/1 -> conv Y/1(coeffsY)
  coeffsX_Top/1 -> conv X1/1(coeffsX)
  coeffsY_Left/1 -> conv Y1/1(coeffsY)
  Abs/1 -> Bit Shift/1
  Abs1/1 -> Bit Shift1/1
  Abs2/1 -> Bit Shift2/1
  Abs3/1 -> Bit Shift3/1
  Abs6/1 -> Bit Shift4/1
  Abs7/1 -> Bit Shift5/1
  Abs8/1 -> Bit Shift6/1
  Abs9/1 -> Bit Shift7/1
  Bit Concat1/1 -> ybypassMux1/3
  Bit Concat2/1 -> ybypassMux/3
  Bit Shift/1 -> Bit Slice/1
  Bit Shift1/1 -> Bit Slice3/1
  Bit Shift2/1 -> Bit Slice2/1
  Bit Shift3/1 -> Bit Slice4/1
  Bit Shift4/1 -> Bit Slice1/1
  Bit Shift5/1 -> Bit Slice6/1
  Bit Shift6/1 -> Bit Slice5/1
  Bit Shift7/1 -> Bit Slice7/1
  Bit Slice/1 -> Sum/1
  Bit Slice1/1 -> Sum2/1
  Bit Slice2/1 -> Sum/2
  Bit Slice3/1 -> Sum1/1
  Bit Slice4/1 -> Sum1/2
  Bit Slice5/1 -> Sum2/2
  Bit Slice6/1 -> Sum3/1
  Bit Slice7/1 -> Sum3/2
  mux/1 -> conv X/2(Image R), conv Y1/2(Image R), conv X1/2(Image R), conv Y/2(Image R)
  mux1/1 -> conv Y/3(Image L), conv X1/3(Image L), conv Y1/3(Image L), conv X/3(Image L)
  Sum/1 -> Sum4/2
  Sum1/1 -> Sum5/2
  Sum2/1 -> Sum4/1
  Sum3/1 -> Sum5/1
  Sum4/1 -> Bit Concat2/1
  Sum5/1 -> Bit Concat1/1
  conv X/1(RX) -> Abs/1
  conv X/2(LX) -> Abs1/1
  conv X1/1(RX) -> Abs6/1
  conv X1/2(LX) -> Abs7/1
  conv Y/1(RY) -> Abs2/1
  conv Y/2(LY) -> Abs3/1
  conv Y1/1(RY) -> Abs8/1
  conv Y1/2(LY) -> Abs9/1
  left_blue/1 -> Bit Concat1/4
  left_green/1 -> Bit Concat1/3
  left_red/1 -> Bit Concat1/2
  right_blue/1 -> Bit Concat2/4
  right_green/1 -> Bit Concat2/3
  right_red/1 -> Bit Concat2/2
  slice left gray/1 -> slicer L operation1/1(channel_in)
  slice right gray/1 -> slicer R operation/1(channel_in)
  slicer L operation1/1(out_1) -> mux1/1
  slicer L operation1/2(out_2) -> mux1/2
  slicer L operation1/3(out_3) -> mux1/3
  slicer L operation1/4(out_4) -> mux1/4
  slicer L operation1/5(out_5) -> mux1/5
  slicer L operation1/6(out_6) -> mux1/6
  slicer L operation1/7(out_7) -> mux1/7
  slicer L operation1/8(out_8) -> mux1/8
  slicer L operation1/9(out_9) -> mux1/9
  slicer R operation/1(out_1) -> mux/1
  slicer R operation/2(out_2) -> mux/2
  slicer R operation/3(out_3) -> mux/3
  slicer R operation/4(out_4) -> mux/4
  slicer R operation/5(out_5) -> mux/5
  slicer R operation/6(out_6) -> mux/6
  slicer R operation/7(out_7) -> mux/7
  slicer R operation/8(out_8) -> mux/8
  slicer R operation/9(out_9) -> mux/9
  ybypassMux/1 -> sobel R_bypass/1, sobel R/1
  sobel R_bypass/1 -> ybypassMux/2
  ybypassMux1/1 -> sobel L_bypass/1, sobel L/1
  sobel L_bypass/1 -> ybypassMux1/2

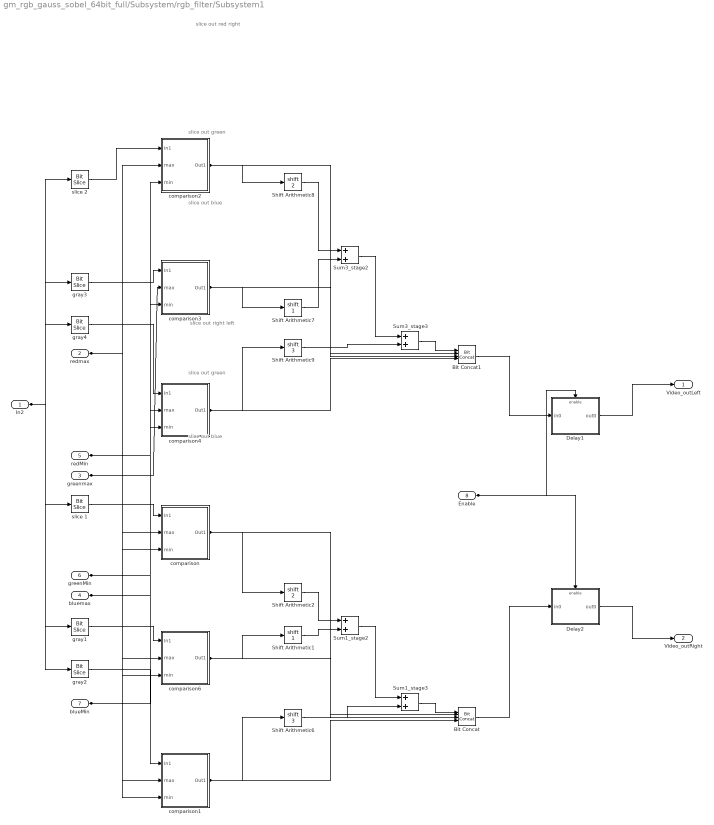
== system gm_rgb_gauss_sobel_64bit_full/Subsystem/rgb_filter/Subsystem1 ==
  note: slice out green
  note: slice out right left
  note: slice out blue
  note: slice out blue
  note: slice out green
  note: slice out red right
  In2 : Inport  OutDataTypeStr=fixdt(0, 64, 0)  PortDimensions=1  SampleTime=2.77039007092199e-06
  redmax : Inport  Port=2  OutDataTypeStr=uint8  PortDimensions=1  SampleTime=2.77039007092199e-06
  greenmax : Inport  Port=3  OutDataTypeStr=uint8  PortDimensions=1  SampleTime=2.77039007092199e-06
  bluemax : Inport  Port=4  OutDataTypeStr=uint8  PortDimensions=1  SampleTime=2.77039007092199e-06
  redMin : Inport  Port=5  OutDataTypeStr=uint8  PortDimensions=1  SampleTime=2.77039007092199e-06
  greenMin : Inport  Port=6  OutDataTypeStr=uint8  PortDimensions=1  SampleTime=2.77039007092199e-06
  blueMin : Inport  Port=7  OutDataTypeStr=uint8  PortDimensions=1  SampleTime=2.77039007092199e-06
  Enable : Inport  Port=8  OutDataTypeStr=boolean  SampleTime=2.77039007092199e-06
  Bit Concat : hdlsllib/Logic and Bit Operations/Bit Concat  numInputs=4
  Bit Concat1 : hdlsllib/Logic and Bit Operations/Bit Concat  numInputs=4
  Delay1 : Subsystem
      settings: MinAlgLoopOccurrences=on
  Delay2 : Subsystem
      settings: MinAlgLoopOccurrences=on
  Shift Arithmetic1 : ArithShift  BitShiftNumber=1  BinPtShiftNumber=double(0)
  Shift Arithmetic2 : ArithShift  BitShiftNumber=2  BinPtShiftNumber=double(0)
  Shift Arithmetic6 : ArithShift  BitShiftNumber=3  BinPtShiftNumber=double(0)
  Shift Arithmetic7 : ArithShift  BitShiftNumber=1  BinPtShiftNumber=double(0)
  Shift Arithmetic8 : ArithShift  BitShiftNumber=2  BinPtShiftNumber=double(0)
  Shift Arithmetic9 : ArithShift  BitShiftNumber=3  BinPtShiftNumber=double(0)
  Sum1_stage2 : Sum  AccumDataTypeStr=uint8  OutDataTypeStr=uint8  SampleTime=2.77039007092199e-06
  Sum1_stage3 : Sum  AccumDataTypeStr=uint8  OutDataTypeStr=uint8  SampleTime=2.77039007092199e-06
  Sum3_stage2 : Sum  AccumDataTypeStr=uint8  OutDataTypeStr=uint8  SampleTime=2.77039007092199e-06
  Sum3_stage3 : Sum  AccumDataTypeStr=uint8  OutDataTypeStr=uint8  SampleTime=2.77039007092199e-06
  comparison : Subsystem
  comparison1 : Subsystem
  comparison2 : Subsystem
  comparison3 : Subsystem
  comparison4 : Subsystem
  comparison6 : Subsystem
  gray1 : hdlsllib/Logic and Bit Operations/Bit Slice  lidx=double(15)  ridx=double(8)
      settings: SourceProductBaseCode=SL
  gray2 : hdlsllib/Logic and Bit Operations/Bit Slice  lidx=double(7)  ridx=double(0)
      settings: SourceProductBaseCode=SL
  gray3 : hdlsllib/Logic and Bit Operations/Bit Slice  lidx=double(47)  ridx=double(40)
      settings: SourceProductBaseCode=SL
  gray4 : hdlsllib/Logic and Bit Operations/Bit Slice  lidx=double(39)  ridx=double(32)
      settings: SourceProductBaseCode=SL
  slice 1 : hdlsllib/Logic and Bit Operations/Bit Slice  lidx=double(23)  ridx=double(16)
      settings: SourceProductBaseCode=SL
  slice 2 : hdlsllib/Logic and Bit Operations/Bit Slice  lidx=double(55)  ridx=double(48)
      settings: SourceProductBaseCode=SL
  Video_outLeft : Outport  SampleTime=2.77039007092199e-06  InitialOutput=0
  Video_outRight : Outport  Port=2  SampleTime=2.77039007092199e-06  InitialOutput=0
  wires:
  Enable/1 -> Delay2/Enable, Delay1/Enable
  In2/1 -> slice 2/1, slice 1/1, gray4/1, gray3/1, gray2/1, gray1/1
  redmax/1 -> comparison2/2(max), comparison/2(max)
  greenmax/1 -> comparison3/2(max), comparison6/2(max)
  bluemax/1 -> comparison4/2(max), comparison1/2(max)
  redMin/1 -> comparison2/3(min), comparison/3(min)
  greenMin/1 -> comparison3/3(min), comparison6/3(min)
  blueMin/1 -> comparison4/3(min), comparison1/3(min)
  Bit Concat/1 -> Delay2/1(in0)
  Bit Concat1/1 -> Delay1/1(in0)
  Delay1/1(out0) -> Video_outLeft/1
  Delay2/1(out0) -> Video_outRight/1
  Shift Arithmetic1/1 -> Sum1_stage2/2
  Shift Arithmetic2/1 -> Sum1_stage2/1
  Shift Arithmetic6/1 -> Sum1_stage3/2
  Shift Arithmetic7/1 -> Sum3_stage2/2
  Shift Arithmetic8/1 -> Sum3_stage2/1
  Shift Arithmetic9/1 -> Sum3_stage3/2
  Sum1_stage3/1 -> Bit Concat/1
  Sum3_stage3/1 -> Bit Concat1/1
  comparison/1(Out1) -> Shift Arithmetic2/1, Bit Concat/2
  comparison1/1(Out1) -> Shift Arithmetic6/1, Bit Concat/4
  comparison2/1(Out1) -> Shift Arithmetic8/1, Bit Concat1/2
  comparison3/1(Out1) -> Shift Arithmetic7/1, Bit Concat1/3
  comparison4/1(Out1) -> Shift Arithmetic9/1, Bit Concat1/4
  comparison6/1(Out1) -> Shift Arithmetic1/1, Bit Concat/3
  gray1/1 -> comparison6/1(In1)
  gray2/1 -> comparison1/1(In1)
  gray3/1 -> comparison3/1(In1)
  gray4/1 -> comparison4/1(In1)
  slice 1/1 -> comparison/1(In1)
  slice 2/1 -> comparison2/1(In1)
  Sum1_stage2/1 -> Sum1_stage3/1
  Sum3_stage2/1 -> Sum3_stage3/1

== system gm_rgb_gauss_sobel_64bit_full/Subsystem/conv_core_gauss/Subsystem1/Delay1 ==
  in0 : Inport  OutDataTypeStr=fixdt(0,16,0,'DataTypeOverride', 'Off')  PortDimensions=[9]  SampleTime=2.77039007092199e-06
  <valid> : EnablePort  OutDataTypeStr=boolean
  Delay1 : Delay  DelayLength=double(1)  InitialCondition=0
  out0 : Outport  OutDataTypeStr=uint16  PortDimensions=[9]  SampleTime=2.77039007092199e-06  InitialOutput=0
  wires:
  Delay1/1 -> out0/1
  in0/1 -> Delay1/1

== system gm_rgb_gauss_sobel_64bit_full/Subsystem/conv_core_gauss/Subsystem1/Delay2 ==
  in0 : Inport  OutDataTypeStr=fixdt(0,16,0,'DataTypeOverride', 'Off')  PortDimensions=[9]  SampleTime=2.77039007092199e-06
  <valid> : EnablePort  OutDataTypeStr=boolean
  Delay2 : Delay  DelayLength=double(1)  InitialCondition=0
  out0 : Outport  OutDataTypeStr=uint16  PortDimensions=[9]  SampleTime=2.77039007092199e-06  InitialOutput=0
  wires:
  Delay2/1 -> out0/1
  in0/1 -> Delay2/1

== system gm_rgb_gauss_sobel_64bit_full/Subsystem/conv_core_gauss/Subsystem1/Delay3 ==
  in0 : Inport  OutDataTypeStr=fixdt(0,32,0,'DataTypeOverride', 'Off')  SampleTime=2.77039007092199e-06
  <valid> : EnablePort  OutDataTypeStr=boolean
  Delay3 : Delay  DelayLength=double(1)  InitialCondition=0
  out0 : Outport  OutDataTypeStr=uint32  SampleTime=2.77039007092199e-06  InitialOutput=0
  wires:
  Delay3/1 -> out0/1
  in0/1 -> Delay3/1

== system gm_rgb_gauss_sobel_64bit_full/Subsystem/conv_core_gauss/Subsystem1/Delay4 ==
  in0 : Inport  OutDataTypeStr=fixdt(0,32,0,'DataTypeOverride', 'Off')  SampleTime=2.77039007092199e-06
  <valid> : EnablePort  OutDataTypeStr=boolean
  Delay4 : Delay  DelayLength=double(1)  InitialCondition=0
  out0 : Outport  OutDataTypeStr=uint32  SampleTime=2.77039007092199e-06  InitialOutput=0
  wires:
  Delay4/1 -> out0/1
  in0/1 -> Delay4/1

== system gm_rgb_gauss_sobel_64bit_full/Subsystem/conv_core_gauss/Subsystem1/Delay5 ==
  in0 : Inport  OutDataTypeStr=fixdt(0,16,0,'DataTypeOverride', 'Off')  PortDimensions=[9]  SampleTime=2.77039007092199e-06
  <valid> : EnablePort  OutDataTypeStr=boolean
  Delay5 : Delay  DelayLength=double(1)  InitialCondition=0
  out0 : Outport  OutDataTypeStr=uint16  PortDimensions=[9]  SampleTime=2.77039007092199e-06  InitialOutput=0
  wires:
  Delay5/1 -> out0/1
  in0/1 -> Delay5/1

== system gm_rgb_gauss_sobel_64bit_full/Subsystem/conv_core_gauss/Subsystem1/Delay6 ==
  in0 : Inport  OutDataTypeStr=fixdt(0,16,0,'DataTypeOverride', 'Off')  PortDimensions=[9]  SampleTime=2.77039007092199e-06
  <valid> : EnablePort  OutDataTypeStr=boolean
  Delay6 : Delay  DelayLength=double(1)  InitialCondition=0
  out0 : Outport  OutDataTypeStr=uint16  PortDimensions=[9]  SampleTime=2.77039007092199e-06  InitialOutput=0
  wires:
  Delay6/1 -> out0/1
  in0/1 -> Delay6/1

== system gm_rgb_gauss_sobel_64bit_full/Subsystem/conv_core_gauss/Subsystem1/Delay7 ==
  in0 : Inport  OutDataTypeStr=fixdt(0,16,0,'DataTypeOverride', 'Off')  PortDimensions=[9]  SampleTime=2.77039007092199e-06
  <valid> : EnablePort  OutDataTypeStr=boolean
  Delay7 : Delay  DelayLength=double(1)  InitialCondition=0
  out0 : Outport  OutDataTypeStr=uint16  PortDimensions=[9]  SampleTime=2.77039007092199e-06  InitialOutput=0
  wires:
  Delay7/1 -> out0/1
  in0/1 -> Delay7/1

== system gm_rgb_gauss_sobel_64bit_full/Subsystem/conv_core_gauss/Subsystem1/Delay8 ==
  in0 : Inport  OutDataTypeStr=fixdt(0,16,0,'DataTypeOverride', 'Off')  PortDimensions=[9]  SampleTime=2.77039007092199e-06
  <valid> : EnablePort  OutDataTypeStr=boolean
  Delay8 : Delay  DelayLength=double(1)  InitialCondition=0
  out0 : Outport  OutDataTypeStr=uint16  PortDimensions=[9]  SampleTime=2.77039007092199e-06  InitialOutput=0
  wires:
  Delay8/1 -> out0/1
  in0/1 -> Delay8/1

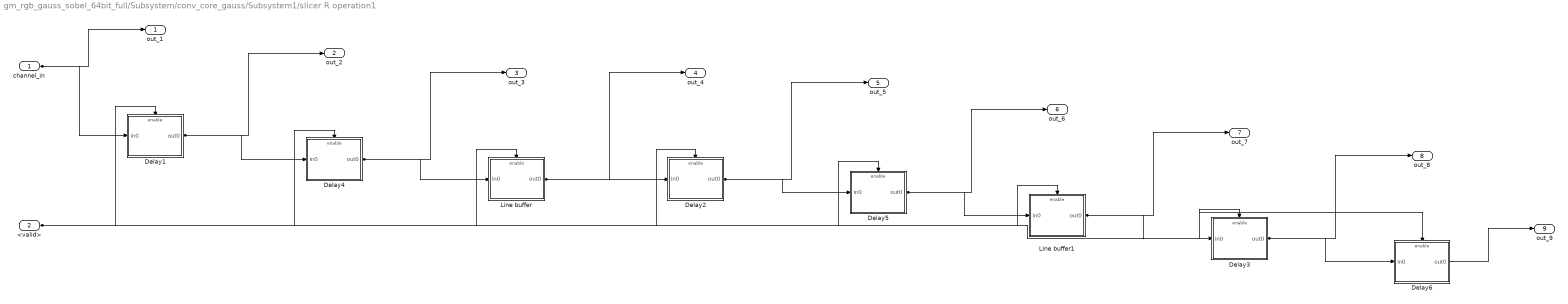
== system gm_rgb_gauss_sobel_64bit_full/Subsystem/conv_core_gauss/Subsystem1/slicer R operation1 ==
  channel_in : Inport  OutDataTypeStr=uint8  PortDimensions=1  SampleTime=2.77039007092199e-06
  <valid> : Inport  Port=2  OutDataTypeStr=boolean  SampleTime=2.77039007092199e-06
  Delay1 : Subsystem
      settings: MinAlgLoopOccurrences=on
  Delay2 : Subsystem
      settings: MinAlgLoopOccurrences=on
  Delay3 : Subsystem
      settings: MinAlgLoopOccurrences=on
  Delay4 : Subsystem
      settings: MinAlgLoopOccurrences=on
  Delay5 : Subsystem
      settings: MinAlgLoopOccurrences=on
  Delay6 : Subsystem
      settings: MinAlgLoopOccurrences=on
  Line buffer : Subsystem
      settings: MinAlgLoopOccurrences=on
  Line buffer1 : Subsystem
      settings: MinAlgLoopOccurrences=on
  out_1 : Outport  SampleTime=2.77039007092199e-06  InitialOutput=0  VectorParamsAs1DForOutWhenUnconnected=off
  out_2 : Outport  Port=2  SampleTime=2.77039007092199e-06  InitialOutput=0  VectorParamsAs1DForOutWhenUnconnected=off
  out_3 : Outport  Port=3  SampleTime=2.77039007092199e-06  InitialOutput=0  VectorParamsAs1DForOutWhenUnconnected=off
  out_4 : Outport  Port=4  SampleTime=2.77039007092199e-06  InitialOutput=0  VectorParamsAs1DForOutWhenUnconnected=off
  out_5 : Outport  Port=5  SampleTime=2.77039007092199e-06  InitialOutput=0  VectorParamsAs1DForOutWhenUnconnected=off
  out_6 : Outport  Port=6  SampleTime=2.77039007092199e-06  InitialOutput=0  VectorParamsAs1DForOutWhenUnconnected=off
  out_7 : Outport  Port=7  SampleTime=2.77039007092199e-06  InitialOutput=0  VectorParamsAs1DForOutWhenUnconnected=off
  out_8 : Outport  Port=8  SampleTime=2.77039007092199e-06  InitialOutput=0  VectorParamsAs1DForOutWhenUnconnected=off
  out_9 : Outport  Port=9  SampleTime=2.77039007092199e-06  InitialOutput=0  VectorParamsAs1DForOutWhenUnconnected=off
  wires:
  channel_in/1 -> Delay1/1(in0), out_1/1
  Delay1/1(out0) -> Delay4/1(in0), out_2/1
  Delay2/1(out0) -> Delay5/1(in0), out_5/1
  Delay3/1(out0) -> Delay6/1(in0), out_8/1
  Delay4/1(out0) -> Line buffer/1(in0), out_3/1
  Delay5/1(out0) -> Line buffer1/1(in0), out_6/1
  Delay6/1(out0) -> out_9/1
  Line buffer/1(out0) -> Delay2/1(in0), out_4/1
  Line buffer1/1(out0) -> Delay3/1(in0), out_7/1
  <valid>/1 -> Line buffer1/Enable, Line buffer/Enable, Delay6/Enable, Delay5/Enable, Delay4/Enable, Delay3/Enable, Delay2/Enable, Delay1/Enable
